simulink model "C_Function_Call_C"  (R2021a)
settings: Solver=FixedStepDiscrete  StartTime=0.0  StopTime=10.0  RelTol=1e-3
CloseFcn:
  | try
  | rmdir slprj\ s
  | catch
  | end
  | try
  | folder_name = [bdroot '*'];
  | rmdir(folder_name,'s')
  | catch
  | end
  | try
  | file_temp_name = [bdroot '.slxc'];
  | delete(file_temp_name)
  | catch
  | end
  | clear folder_name file_temp_name
settings Model: Creator=jetson  LastModifiedBy=jetson
settings DataIOCC: SaveOutput=off  SignalLogging=off  DSMLogging=off  SaveTime=off  ReturnWorkspaceOutputs=off
settings OptimizationCC: DefaultParameterBehavior=Inlined  EnhancedBackFolding=on  PassReuseOutputArgsAs=Individual arguments  ZeroExternalMemoryAtStartup=off  ZeroInternalMemoryAtStartup=off  OptimizeBlockOrder=speed  DifferentSizesBufferReuse=on  OptimizationCustomize=off  EfficientTunableParamExpr=on
settings DebuggingCC: ParameterTunabilityLossMsg=error
settings SFSimCC: SimCustomHeaderCode="#include \"data_array.h\""  SimUserSources=data_array.c  MATLABDynamicMemAlloc=off
settings RTWCC: SystemTargetFile=ert.tlc  GenCodeOnly=on  TemplateMakefile=ert_default_tmf  GenerateReport=on  RTWUseSimCustomCode=on  CustomHeaderCode="#include \"data_array.h\""  CustomSource=data_array.c  IncludeHyperlinkInReport=on  LaunchReport=on  GenerateTraceInfo=on
settings CodeAppCC: ForceParamTrailComments=on  IgnoreCustomStorageClasses=off  OperatorAnnotations=on  SimulinkDataObjDesc=on  SFDataObjDesc=on  InsertBlockDesc=on
settings ERTTargetCC: TargetLangStandard=C99 (ISO)  GenerateSampleERTMain=on  InlinedParameterPlacement=NonHierarchical  ERTCustomFileTemplate=example_file_process.tlc

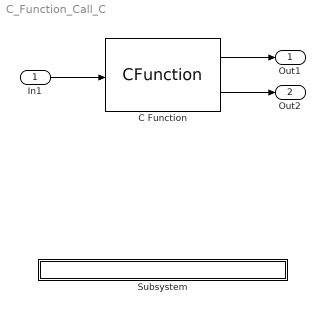
== system C_Function_Call_C ==
  In1 : Inport  PortDimensions=100
      settings: AttributesFormatString=Data Type : %<OutDataTypeStr>
  C Function : CFunction  OutputCode=|
      | /* declare the struct dataArr */
      | DataArray dataArr;
      | /* store the length and data coming in from the input port */
      | dataArr.pData = &data[0];
      | dataArr.length = length;
      | 
      | /* call the function from the external code to calculate sum */
      | sum = data_sum(dataArr);
      | 
      | /* calculate the mean */
      | mean = sum / length;
      settings: AttributesFormatString=%<OutputCode>
  Subsystem : Subsystem
      settings: OpenFcn=web(fullfile(docroot, 'simulink/ug/call-and-integrate-external-c-algorithms-into-simulink.html'))
      mask Display: disp('double click open help')
  Out1 : Outport
      settings: AttributesFormatString=Data Type : %<OutDataTypeStr>
  Out2 : Outport  Port=2
      settings: AttributesFormatString=Data Type : %<OutDataTypeStr>
  wires:
  In1/1 -> C Function/1
  C Function/1 -> Out1/1
  C Function/2 -> Out2/1

== system C_Function_Call_C/Subsystem ==
